simulink model "MotorSim"  (R2018a)
settings: Solver=VariableStepAuto  StartTime=0.0  StopTime=1  MaxStep=1/(PWM_Resolution*PWM_Frequency)  RelTol=1e-3
PreLoadFcn:
  | modelDir = fileparts(get_param(bdroot, 'FileName'));
  | addpath(fullfile(modelDir,'Parameters'));
  | addpath(fullfile(modelDir,'subsystems'));
  | 
  | Parameters_Model
  | Parameters_Simulation
  | Parameters_Controller
InitFcn:
  | Parameters_Model
  | Parameters_Simulation
  | Parameters_Controller
undefined symbols (not defined in the file): PWM_Duty, PWM_Frequency, PWM_Resolution
libraries: simulink x4
settings Model: Creator=Thomas  LastModifiedBy=Thomas

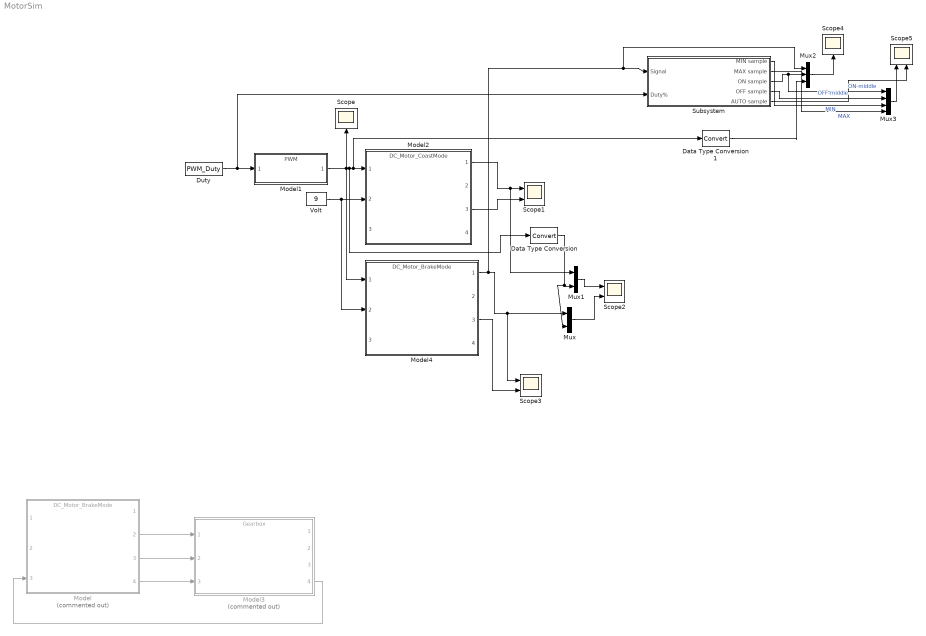
== system MotorSim ==
  Data Type Conversion : DataTypeConversion  RndMeth=Round
  Data Type Conversion1 : DataTypeConversion  RndMeth=Round
  Duty : Constant  Value=PWM_Duty
  Model : ModelReference  Commented=on  ModelNameDialog=DC_Motor_BrakeMode  SimulationMode=Normal  ModelReferenceVersion=1.14
  Model1 : ModelReference  ModelNameDialog=PWM  SimulationMode=Normal  ModelReferenceVersion=1.19
  Model2 : ModelReference  ModelNameDialog=DC_Motor_CoastMode  SimulationMode=Normal  ModelReferenceVersion=1.30
  Model3 : ModelReference  Commented=on  ModelNameDialog=Gearbox  SimulationMode=Normal  ModelReferenceVersion=1.7
  Model4 : ModelReference  ModelNameDialog=DC_Motor_BrakeMode  SimulationMode=Normal  ModelReferenceVersion=1.14
  Mux : Mux  Inputs=2
  Mux1 : Mux  Inputs=2
  Mux2 : Mux  Inputs=3
  Mux3 : Mux
  Scope : Scope
  Scope{1..3,5} (4 alike) : Scope  NumInputPorts=2
  Scope4 : Scope
  Subsystem : Subsystem
  Volt : Constant  Value=9
  wires:
  Volt/1 -> Model4/2, Model2/2
  Duty/1 -> Subsystem/2(Duty%), Model1/1
  Model3/4 -> Model/3
  Model/4 -> Model3/3
  Model/3 -> Model3/2
  Model/2 -> Model3/1
  Model2/3 -> Scope1/2
  Model4/1 -> Mux2/1, Subsystem/1(Signal), Scope3/1, Mux/1
  Mux/1 -> Scope2/2
  Mux1/1 -> Scope2/1
  Model1/1 -> Model4/1, Data Type Conversion/1, Data Type Conversion1/1, Model2/1, Scope/1
  Data Type Conversion/1 -> Mux/2, Mux1/2
  Model4/3 -> Scope3/2
  Model2/1 -> Mux1/1, Scope1/1
  Mux2/1 -> Scope4/1
  Data Type Conversion1/1 -> Mux2/3
  Subsystem/3(ON sample) -> Mux3/1, Mux2/2  "ON-middle"
  Mux3/1 -> Scope5/1
  Subsystem/4(OFF sample) -> Mux3/2  "OFF-middle"
  Subsystem/5(AUTO sample) -> Scope5/2
  Subsystem/1(MIN sample) -> Mux3/3  "MIN"
  Subsystem/2(MAX sample) -> Mux3/4  "MAX"

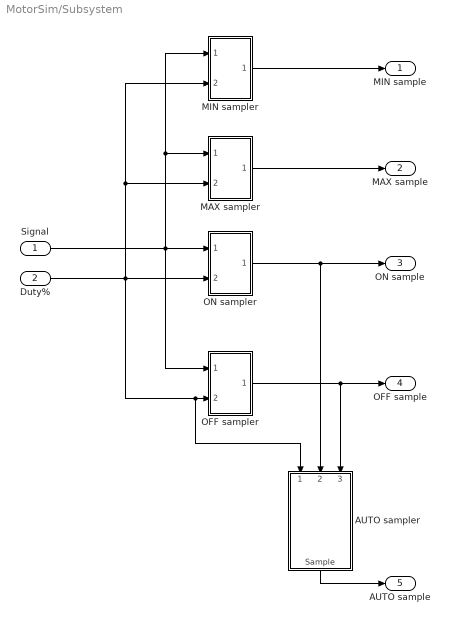
== system MotorSim/Subsystem ==
  Signal : Inport
  Duty% : Inport  Port=2  OutDataTypeStr=double
  AUTO sampler : Subsystem
  MAX sampler : Subsystem
  MIN sampler : Subsystem
  OFF sampler : Subsystem
  ON sampler : Subsystem
  MIN sample : Outport
  MAX sample : Outport  Port=2
  ON sample : Outport  Port=3
  OFF sample : Outport  Port=4
  AUTO sample : Outport  Port=5
  wires:
  Signal/1 -> MAX sampler/1(Signal), MIN sampler/1(Signal), OFF sampler/1(Signal), ON sampler/1(Signal)
  ON sampler/1(Sample) -> AUTO sampler/2(ON sample), ON sample/1
  OFF sampler/1(Sample) -> AUTO sampler/3(OFF sample), OFF sample/1
  AUTO sampler/1(Sample) -> AUTO sample/1
  Duty%/1 -> MIN sampler/2(Duty%), MAX sampler/2(Duty%), AUTO sampler/1(Duty%), OFF sampler/2(Duty%), ON sampler/2(Duty%)
  MAX sampler/1(Sample) -> MAX sample/1
  MIN sampler/1(Sample) -> MIN sample/1

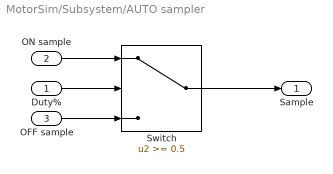
== system MotorSim/Subsystem/AUTO sampler ==
  Duty% : Inport  OutDataTypeStr=double
  ON sample : Inport  Port=2
  OFF sample : Inport  Port=3
  Switch : Switch  Threshold=0.5
  Sample : Outport
  wires:
  Duty%/1 -> Switch/2
  ON sample/1 -> Switch/1
  OFF sample/1 -> Switch/3
  Switch/1 -> Sample/1

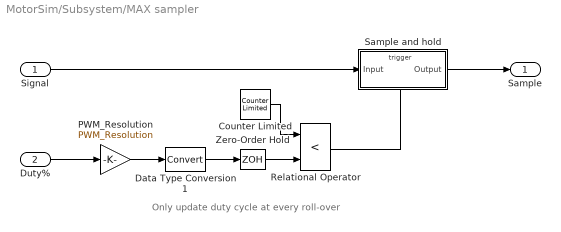
== system MotorSim/Subsystem/MAX sampler ==
  note: Only update duty cycle at every roll-over
  Signal : Inport
  Duty% : Inport  Port=2  OutDataTypeStr=double
  Counter Limited : simulink/Sources/Counter Limited  uplimit=PWM_Resolution-1  tsamp=1/(PWM_Resolution*PWM_Frequency)
  Data Type Conversion1 : DataTypeConversion  RndMeth=Round
  PWM_Resolution : Gain  Gain=PWM_Resolution
  Relational Operator : RelationalOperator  Operator=<  OutDataTypeStr=boolean  RndMeth=Simplest
  Sample and hold : Subsystem
  Zero-Order Hold : ZeroOrderHold  SampleTime=1/PWM_Frequency
  Sample : Outport
  wires:
  Relational Operator/1 -> Sample and hold/Trigger
  Zero-Order Hold/1 -> Relational Operator/2
  Counter Limited/1 -> Relational Operator/1
  Signal/1 -> Sample and hold/1(Input)
  Data Type Conversion1/1 -> Zero-Order Hold/1
  PWM_Resolution/1 -> Data Type Conversion1/1
  Sample and hold/1(Output) -> Sample/1
  Duty%/1 -> PWM_Resolution/1

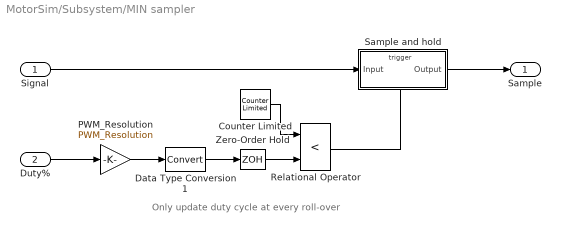
== system MotorSim/Subsystem/MIN sampler ==
  note: Only update duty cycle at every roll-over
  Signal : Inport
  Duty% : Inport  Port=2  OutDataTypeStr=double
  Counter Limited : simulink/Sources/Counter Limited  uplimit=PWM_Resolution-1  tsamp=1/(PWM_Resolution*PWM_Frequency)
  Data Type Conversion1 : DataTypeConversion  RndMeth=Round
  PWM_Resolution : Gain  Gain=PWM_Resolution
  Relational Operator : RelationalOperator  Operator=<  OutDataTypeStr=boolean  RndMeth=Simplest
  Sample and hold : Subsystem
  Zero-Order Hold : ZeroOrderHold  SampleTime=1/PWM_Frequency
  Sample : Outport
  wires:
  Relational Operator/1 -> Sample and hold/Trigger
  Zero-Order Hold/1 -> Relational Operator/2
  Counter Limited/1 -> Relational Operator/1
  Signal/1 -> Sample and hold/1(Input)
  Data Type Conversion1/1 -> Zero-Order Hold/1
  PWM_Resolution/1 -> Data Type Conversion1/1
  Sample and hold/1(Output) -> Sample/1
  Duty%/1 -> PWM_Resolution/1

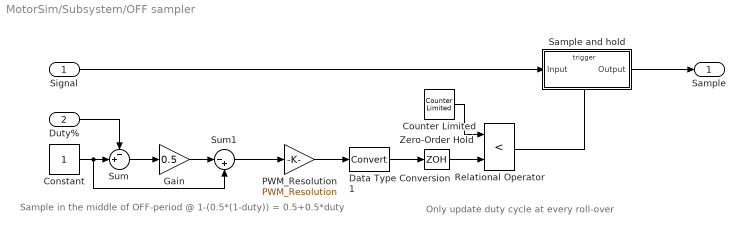
== system MotorSim/Subsystem/OFF sampler ==
  note: Sample in the middle of OFF-period @ 1-(0.5*(1-duty)) = 0.5+0.5*duty
  note: Only update duty cycle at every roll-over
  Signal : Inport
  Duty% : Inport  Port=2  OutDataTypeStr=double
  Constant : Constant
  Counter Limited : simulink/Sources/Counter Limited  uplimit=PWM_Resolution-1  tsamp=1/(PWM_Resolution*PWM_Frequency)
  Data Type Conversion1 : DataTypeConversion  RndMeth=Round
  Gain : Gain  Gain=0.5
  PWM_Resolution : Gain  Gain=PWM_Resolution
  Relational Operator : RelationalOperator  Operator=<  OutDataTypeStr=boolean  RndMeth=Simplest
  Sample and hold : Subsystem
  Sum : Sum  Inputs=-+|
  Sum1 : Sum  Inputs=|-+
  Zero-Order Hold : ZeroOrderHold  SampleTime=1/PWM_Frequency
  Sample : Outport
  wires:
  Relational Operator/1 -> Sample and hold/Trigger
  Zero-Order Hold/1 -> Relational Operator/2
  Counter Limited/1 -> Relational Operator/1
  Signal/1 -> Sample and hold/1(Input)
  Duty%/1 -> Sum/1
  Data Type Conversion1/1 -> Zero-Order Hold/1
  PWM_Resolution/1 -> Data Type Conversion1/1
  Sample and hold/1(Output) -> Sample/1
  Sum/1 -> Gain/1
  Constant/1 -> Sum1/2, Sum/2
  Gain/1 -> Sum1/1
  Sum1/1 -> PWM_Resolution/1

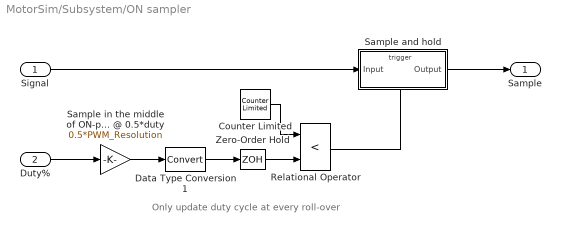
== system MotorSim/Subsystem/ON sampler ==
  note: Only update duty cycle at every roll-over
  Signal : Inport
  Duty% : Inport  Port=2  OutDataTypeStr=double
  Counter Limited : simulink/Sources/Counter Limited  uplimit=PWM_Resolution-1  tsamp=1/(PWM_Resolution*PWM_Frequency)
  Data Type Conversion1 : DataTypeConversion  RndMeth=Round
  Relational Operator : RelationalOperator  Operator=<  OutDataTypeStr=boolean  RndMeth=Simplest
  Sample and hold : Subsystem
  Sample in the middle of ON-period @ 0.5*duty : Gain  Gain=0.5*PWM_Resolution
  Zero-Order Hold : ZeroOrderHold  SampleTime=1/PWM_Frequency
  Sample : Outport
  wires:
  Relational Operator/1 -> Sample and hold/Trigger
  Zero-Order Hold/1 -> Relational Operator/2
  Counter Limited/1 -> Relational Operator/1
  Signal/1 -> Sample and hold/1(Input)
  Data Type Conversion1/1 -> Zero-Order Hold/1
  Sample in the middle of ON-period @ 0.5*duty/1 -> Data Type Conversion1/1
  Sample and hold/1(Output) -> Sample/1
  Duty%/1 -> Sample in the middle of ON-period @ 0.5*duty/1

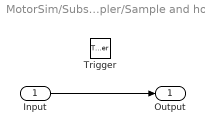
== system MotorSim/Subsystem/MAX sampler/Sample and hold ==
  Input : Inport
  Trigger : TriggerPort  TriggerType=falling  VariantControl=Variant  PortDimensions=1
  Output : Outport
  wires:
  Input/1 -> Output/1

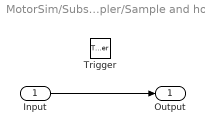
== system MotorSim/Subsystem/MIN sampler/Sample and hold ==
  Input : Inport
  Trigger : TriggerPort  VariantControl=Variant  PortDimensions=1
  Output : Outport
  wires:
  Input/1 -> Output/1

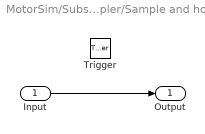
== system MotorSim/Subsystem/OFF sampler/Sample and hold ==
  Input : Inport
  Trigger : TriggerPort  TriggerType=falling  VariantControl=Variant  PortDimensions=1
  Output : Outport
  wires:
  Input/1 -> Output/1

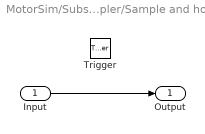
== system MotorSim/Subsystem/ON sampler/Sample and hold ==
  Input : Inport
  Trigger : TriggerPort  TriggerType=falling  VariantControl=Variant  PortDimensions=1
  Output : Outport
  wires:
  Input/1 -> Output/1
